simulink model "trigonometry_model"  (R2021b)
settings: Solver=VariableStepAuto  StartTime=0.0  StopTime=1  RelTol=1e-3
settings Model: Creator=Bhumil Depani  LastModifiedBy=Bhumil Depani

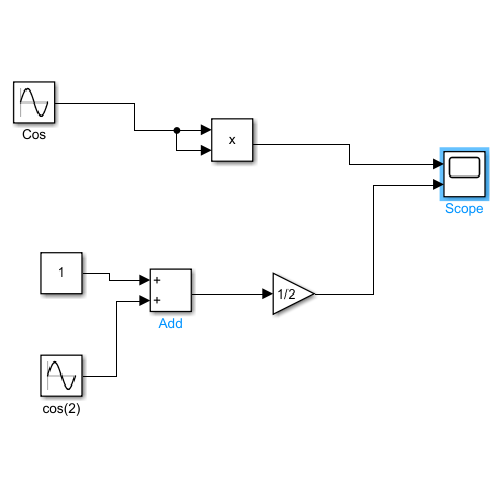
[thumbnail: Simulink's stored preview of the top-level diagram]
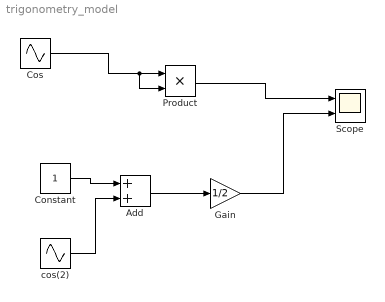
== system trigonometry_model ==
  Add : Sum
  Constant : Constant
  Cos : Sin  Frequency=2*pi*1  Phase=pi/2  SampleTime=0
  Gain : Gain  Gain=1/2
  Product : Product
  Scope : Scope  NumInputPorts=2
  cos(2) : Sin  Frequency=2*pi*1*2  Phase=pi/2  SampleTime=0
  wires:
  Product/1 -> Scope/1
  Constant/1 -> Add/1
  cos(2)/1 -> Add/2
  Add/1 -> Gain/1
  Gain/1 -> Scope/2
  Cos/1 -> Product/2, Product/1
